simulink model "input_signal"  (R2013a)
settings: Solver=VariableStepDiscrete  StartTime=0.0  StopTime=10.0  MaxStep=0.0001  RelTol=1e-3
settings Model: Creator=Vittorio  LastModifiedBy=s171105
settings OptimizationCC: ExpressionDepthLimit=2147483647
settings DebuggingCC: StrictBusMsg=Warning
settings GRTTargetCC: CombineOutputUpdateFcns=off  GRTInterface=on

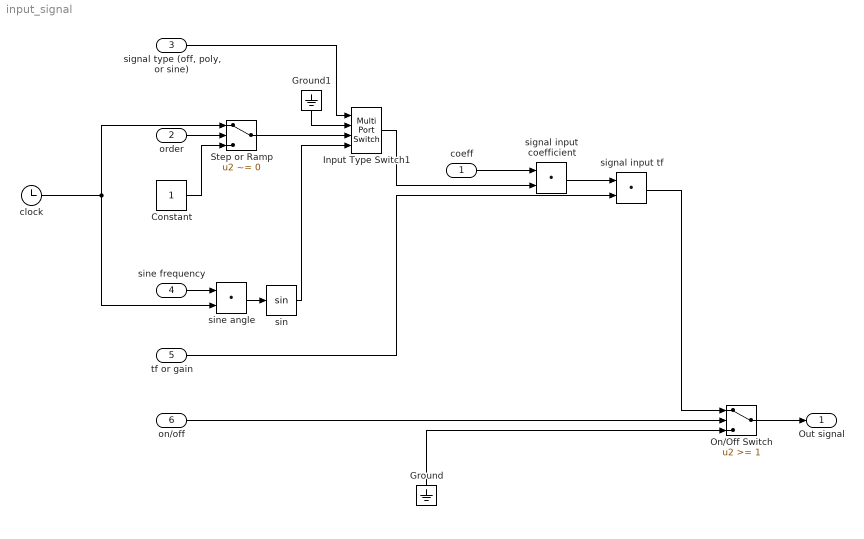
== system input_signal ==
  coeff : Inport
  order : Inport  Port=2
  "signal type (off, poly, or sine)" : Inport  Port=3
  sine frequency : Inport  Port=4
  tf or gain : Inport  Port=5
  on/off : Inport  Port=6
  Constant : Constant
  Ground : Ground
  Ground1 : Ground
  Input Type Switch1 : MultiPortSwitch  DataPortOrder=Zero-based contiguous  zeroidx=on
  On/Off Switch : Switch  Threshold=1
  Step or Ramp : Switch  Criteria=u2 ~= 0  Threshold=1
  clock : Clock
  signal input coefficient : DotProduct  InputSameDT=on  OutDataTypeStr=Inherit: Inherit via internal rule
  signal input tf : DotProduct  InputSameDT=on  OutDataTypeStr=Inherit: Inherit via internal rule
  sin : Trigonometry
  sine angle : DotProduct  InputSameDT=on  OutDataTypeStr=Inherit: Inherit via internal rule
  Out signal : Outport
  wires:
  Ground/1 -> On/Off Switch/3
  on/off/1 -> On/Off Switch/2
  On/Off Switch/1 -> Out signal/1
  sine angle/1 -> sin/1
  sine frequency/1 -> sine angle/1
  sin/1 -> Input Type Switch1/4
  order/1 -> Step or Ramp/2
  coeff/1 -> signal input coefficient/1
  Input Type Switch1/1 -> signal input coefficient/2
  "signal type (off, poly, or sine)"/1 -> Input Type Switch1/1
  Ground1/1 -> Input Type Switch1/2
  Step or Ramp/1 -> Input Type Switch1/3
  signal input coefficient/1 -> signal input tf/1
  tf or gain/1 -> signal input tf/2
  signal input tf/1 -> On/Off Switch/1
  clock/1 -> sine angle/2, Step or Ramp/1
  Constant/1 -> Step or Ramp/3
